simulink model "incremental_simplePseudoinverse"  (R2017a)
settings: Solver=VariableStepAuto  StartTime=0.0  StopTime=10.0  RelTol=1e-3
settings Model: Creator=Luca  LastModifiedBy=Luca

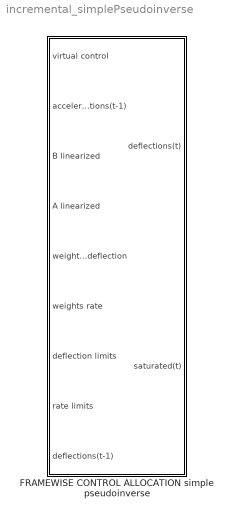
== system incremental_simplePseudoinverse ==
  FRAMEWISE CONTROL ALLOCATION simple pseudoinverse : Subsystem

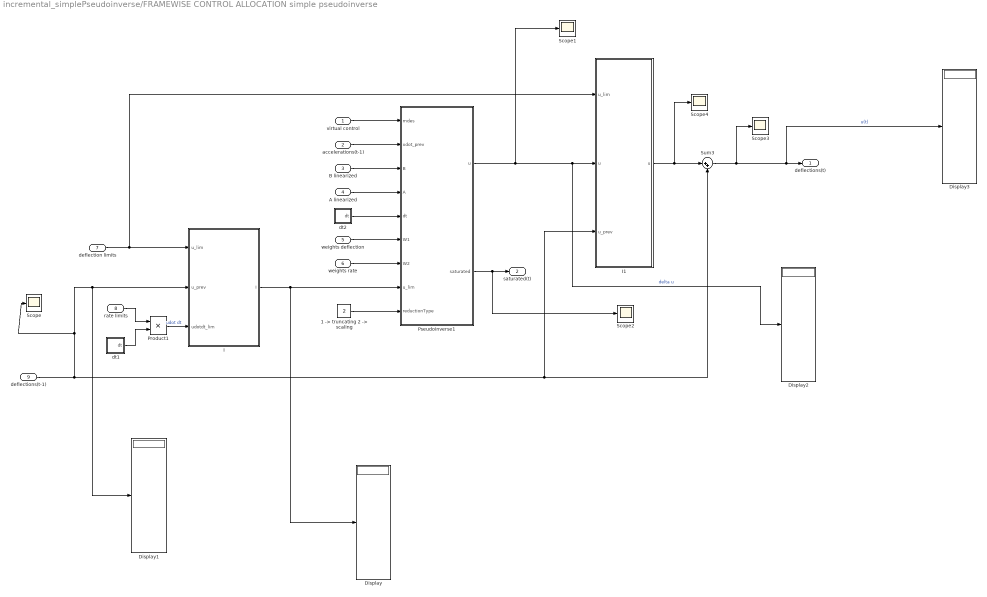
== system incremental_simplePseudoinverse/FRAMEWISE CONTROL ALLOCATION simple pseudoinverse ==
  virtual control : Inport
  "accelerations(t-1) " : Inport  Port=2
  B linearized : Inport  Port=3
  A linearized : Inport  Port=4
  weights deflection : Inport  Port=5
  weights rate : Inport  Port=6
  deflection limits : Inport  Port=7
  rate limits : Inport  Port=8
  deflections(t-1) : Inport  Port=9
  "1 -> truncating 2 -> scaling" : Constant  Value=2
  Display{,1..3} (4 alike) : Display
  I : MATLAB Function  TreatAsAtomicUnit=on
  I1 : MATLAB Function  TreatAsAtomicUnit=on
  Product1 : Product
  Pseudoinverse1 : MATLAB Function  TreatAsAtomicUnit=on
  Scope{,1..4} (5 alike) : Scope
  Sum3 : Sum  Inputs=|++
  dt1 : Subsystem
  dt2 : Subsystem
  deflections(t) : Outport
  saturated(t) : Outport  Port=2
  wires:
  I/1(I) -> Display/1, Pseudoinverse1/8(u_lim)
  Product1/1 -> I/3(udotdt_lim)  "udot dt"
  rate limits/1 -> Product1/1
  deflection limits/1 -> I/1(u_lim), I1/1(u_lim)
  weights deflection/1 -> Pseudoinverse1/6(W1)
  "1 -> truncating 2 -> scaling"/1 -> Pseudoinverse1/9(reductionType)
  virtual control/1 -> Pseudoinverse1/1(mdes)
  dt2/1(dt) -> Pseudoinverse1/5(dt)
  A linearized/1 -> Pseudoinverse1/4(A)
  dt1/1(dt) -> Product1/2
  Pseudoinverse1/2(saturated) -> Scope2/1, saturated(t)/1
  deflections(t-1)/1 -> Sum3/2, I1/3(u_prev), Display1/1, I/2(u_prev), Scope/1
  I1/1(u) -> Scope4/1, Sum3/1
  Pseudoinverse1/1(u) -> Scope1/1, Display2/1, I1/2("u ")  "delta u"
  Sum3/1 -> Scope3/1, Display3/1, deflections(t)/1  "u(t)"
  B linearized/1 -> Pseudoinverse1/3(B)
  weights rate/1 -> Pseudoinverse1/7(W2)
  "accelerations(t-1) "/1 -> Pseudoinverse1/2(xdot_prev)

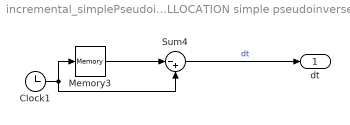
== system incremental_simplePseudoinverse/FRAMEWISE CONTROL ALLOCATION simple pseudoinverse/dt1 ==
  Clock1 : Clock
  Memory3 : Memory
  Sum4 : Sum  Inputs=|-+
  dt : Outport
  wires:
  Clock1/1 -> Sum4/2, Memory3/1
  Memory3/1 -> Sum4/1
  Sum4/1 -> dt/1  "dt"

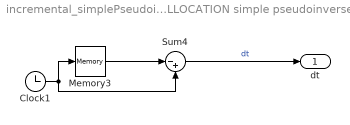
== system incremental_simplePseudoinverse/FRAMEWISE CONTROL ALLOCATION simple pseudoinverse/dt2 ==
  Clock1 : Clock
  Memory3 : Memory
  Sum4 : Sum  Inputs=|-+
  dt : Outport
  wires:
  Clock1/1 -> Sum4/2, Memory3/1
  Memory3/1 -> Sum4/1
  Sum4/1 -> dt/1  "dt"

== matlab function incremental_simplePseudoinverse/FRAMEWISE CONTROL ALLOCATION simple pseudoinverse/I ==
  data: u_lim input; u_prev input; udotdt_lim input; I output
function I = computeIntersection(u_lim, u_prev, udotdt_lim)
%check if the matrices are correct
    if not(isequal(size(u_lim,1),size(udotdt_lim,1), size(u_prev,1)))
        error ('input matrix dimensions do not match')
    end

%declare space of intersection
    I = zeros(length(u_lim),2);
    
    I(:,1) = max(-udotdt_lim, u_lim(:,1)-u_prev);
    I(:,2) = min(+udotdt_lim, u_lim(:,2)-u_prev);
    
end

== matlab function incremental_simplePseudoinverse/FRAMEWISE CONTROL ALLOCATION simple pseudoinverse/I1 ==
  data: u_lim input; u input; u output; u_prev input
function u = uCheck(u_lim, u, u_prev)
%check if the matrices are correct
    if not(isequal(size(u_lim,1), size(u,1)))
        error ('input matrix dimensions do not match')
    end

%if computation error occur, correct deflections
    for i = 1:length(u)
        if u(i)+u_prev(i) > u_lim(i,2)
            u(i) = u_lim(i,2)-u_prev(i);
        end
        if u(i)+u_prev(i) < u_lim(i,1)
            u(i) = u_lim(i,1)-u_prev(i);
        end    
    
end

== matlab function incremental_simplePseudoinverse/FRAMEWISE CONTROL ALLOCATION simple pseudoinverse/Pseudoinverse1 ==
  data: mdes input; xdot_prev input; u output; B input; A input; dt input; W1 input; W2 input; u_lim input; reductionType input; saturated output
function [u, saturated] = Pseudoinverse(mdes, xdot_prev, B, A, dt, W1, W2, u_lim, reductionType)
coder.varsize('u_index', 'Br', 'Wr', 'u_sat');

%check if the matrices are correct
    if not(isequal(size(u_lim,1),size(B,2),size(W1,1),size(W1,2),size(W2,1),size(W2,2))...
       && isequal(size(mdes,1),size(B,1),size(A,1),size(A,2),size(xdot_prev,1)))
        error ('input matrix dimensions do not match')
    end
    
%assign to every equation an index    
    I = eye(length(xdot_prev));
    
%compute the remaining moment to compensate
    m = mdes - (I + A*dt)*xdot_prev;
    
%check the type of system and then compute the pseudoinverse 1st step
    order = size(B,2)-size(B,1);

    if order > 0 %over-determined, solution that minimizes the 2norm
        u = inv(W1)*B'*inv(B*inv(W1)*B')*m;
%             W = power((power(W1,2) + power(W2,2)),1/2);
%             H = B*inv(W);
%             G = inv(W) * (H'*inv(H*H'));
%             II = eye(size(G*B,1));
%             F = (II - G*B)*power(inv(W),2)*power(W2,2);
%             u = inv(W)*B'*inv(B*inv(W)*B')*m;
    elseif order < 0 %under-determined, solution that minimizes the error
        u = inv(B'*B)*B'*m;   
    else %order = 0, sqared thus invertiBrle
        u = inv(B)*m;
    end

%deifne u_sat vector
    u_sat = zeros(length(u),1);
    
    saturated = 0;
%check if the first iteration solution is correct then return    
    if not(any(u <= u_lim(:,1))||any(u >= u_lim(:,2)))  
        return
    end
    
    saturated = 1;
%The software continues only if the solution has to be reduced
%reduce their value
    switch reductionType
        case 1 %truncation
            %takes note of which one are out of their bounds
                u_sat(u < u_lim(:,1)) = 1;
                u_sat(u > u_lim(:,2)) = 1;
                
            %trucate
                u = min(u, u_lim(:,2));
                u = max(u, u_lim(:,1));

        case 2 %scaling solution -> direction preserving
            %reduce
                a = zeros(length(u),1);

                for i = 1:length(u)
                    if u(i)>0
                       a(i) = abs(u(i)/u_lim(i,2));
                    elseif u(i)<0
                       a(i) = abs(u(i)/u_lim(i,1));
                    else
                       a(i) = 0; 
                    end          
                end
                a_max = max(a);
                a_max = max(a_max,1);
                u = u/a_max;
            
            %takes note of which one are out of their bounds
                u_sat(u == u_lim(:,2)) = 1;
                u_sat(u == u_lim(:,1)) = 1;
            
    end
    
return
    
end
